simulink model "verify_CondensingBoiler_mdl"  (R2013b)
settings: Solver=ode45  StartTime=0.0  StopTime=1800  MaxStep=10  RelTol=1e-3
libraries: carnot x3, simulink x1
settings Model: Creator=drhf  LastModifiedBy=drhf
settings DataIOCC: LimitDataPoints=off
settings OptimizationCC: ExpressionDepthLimit=2147483647
settings DebuggingCC: StateNameClashWarn=warning
settings GRTTargetCC: CombineOutputUpdateFcns=off  GRTInterface=on

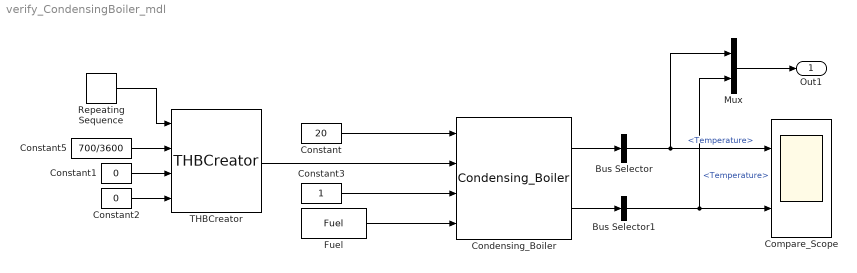
== system verify_CondensingBoiler_mdl ==
  Bus Selector : BusSelector  OutputSignals=Temperature
  Bus Selector1 : BusSelector  OutputSignals=THBin.Temperature
  Compare_Scope : Scope  NumInputPorts=2
      settings: YMin=-5~-5  YMax=5~5
  Condensing_Boiler : carnot/Source/Boiler/Condensing_Boiler  Pnom=20e3  U=3  vol=0.02  electricPower=[20 120]  relativeQdot=[0.25 1]  whichTforEfficiency=mean of inlet and outlet temperature  temperatures="[40  70]"  efficiency=[1.05 0.95; 1.0 0.9]  lin=10  qua=100  Tini=20  nodes=1
  Constant : Constant  Value=20
  Constant1 : Constant  Value=0
  Constant2 : Constant  Value=0
  Constant3 : Constant
  Constant5 : Constant  Value=700/3600
  Fuel : carnot/Source/Energy/Fuel  ft=1  t=20  ls=3.5  p=1.013e5  h_values=[5.14e7 5.69e7]  tc=45  price=1  mass=[0.33 0.67 0 0 0 0]
  Mux : Mux  Inputs=2
  Repeating Sequence : simulink/Sources/Repeating Sequence  rep_seq_t="[0 200  1500 1801]"  rep_seq_y=[30 30 65 65]
  THBCreator : carnot/Basic/Hydraulics/THBCreator  Inport_ID=off  Inport_T=on  Inport_mdot=on  Inport_p=off  Inport_type=off  Inport_mix=off  Inport_mix2=on  Inport_mix3=on  Inport_d=off  Inport_c=off  Inport_l=off  Inport_q=off  Inport_LH=off  Inport_H=off  ID=20001  T=30  mdot=0  p=2e5  FluidType=1  FluidMix=0  FluidMix2=0  FluidMix3=0  d=0.02  c=0  l=0  q=0  LH=0  H=0  Annotation_ID=off  Annotation_T=off  Annotation_mdot=off  Annotation_p=off  Annotation_type=off  Annotation_mix=off  Annotation_mix2=off  Annotation_mix3=off  Annotation_d=off  Annotation_c=off  Annotation_l=off  Annotation_q=off  Annotation_LH=off  Annotation_H=off
  Out1 : Outport
  wires:
  Condensing_Boiler/1 -> Bus Selector/1
  Bus Selector/1 -> Mux/1, Compare_Scope/1  "<Temperature>"
  Condensing_Boiler/2 -> Bus Selector1/1
  Bus Selector1/1 -> Mux/2, Compare_Scope/2  "<Temperature>"
  Mux/1 -> Out1/1
  Constant5/1 -> THBCreator/2
  Repeating Sequence/1 -> THBCreator/1
  Constant/1 -> Condensing_Boiler/1
  THBCreator/1 -> Condensing_Boiler/2
  Fuel/1 -> Condensing_Boiler/4
  Constant3/1 -> Condensing_Boiler/3
  Constant1/1 -> THBCreator/3
  Constant2/1 -> THBCreator/4
